simulink model "Pitch_Velocity_Controllers_Jetstar_FC4_Testing_Linear_Model"  (R2020a)
settings: Solver=FixedStepAuto  StartTime=0.0  StopTime=300  FixedStep=0.01  RelTol=1e-3
values from neighbouring files (symbols this model uses):
  A_Long = [Xu                     , Xw                      , -w_0                         , -g*cos(theta_0) ... (first row only)    [Longitudinal_Linearized_Matrices.m]
  B_Long = [Xdel_e                          , Xdel_t ... (first row only)    [Longitudinal_Linearized_Matrices.m]
  C_Long = eye(4)    [Longitudinal_Linearized_Matrices.m]
  D_Long = zeros(4,2)    [Longitudinal_Linearized_Matrices.m]
undefined symbols (not defined in the file or in its folder): theta_0, u_0, w_0, z_0
libraries: cstblocks x3, simulink_extras x1
settings Model: Creator=mohan  LastModifiedBy=mohan

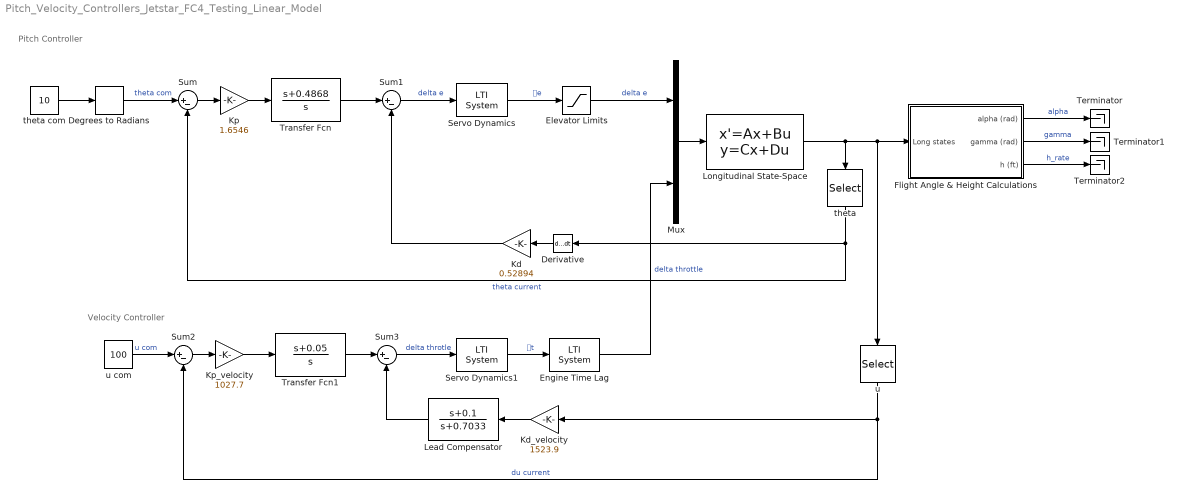
== system Pitch_Velocity_Controllers_Jetstar_FC4_Testing_Linear_Model ==
  note: Velocity Controller
  note: Pitch Controller
  Degrees to Radians : simulink_extras/Transformations/Degrees to Radians
  Derivative : Derivative
  Elevator Limits : Saturate  UpperLimit=25*pi/180  LowerLimit=-25*pi/180
  Engine Time Lag : cstblocks/LTI System  sys=tf(0.1,[1 0.1])  IC=[]
  Flight Angle & Height Calculations : Subsystem
  Kd : Gain  Gain=0.52894
  Kd_velocity : Gain  Gain=1523.9
  Kp : Gain  Gain=1.6546
  Kp_velocity : Gain  Gain=1027.7
  Lead Compensator : TransferFcn  Numerator=[1 0.1]  Denominator=[1 0.7033]
  Longitudinal State-Space : StateSpace  A=A_Long  B=B_Long  C=C_Long  D=D_Long  InitialCondition=[]
  Mux : Mux  Inputs=2
  Servo Dynamics : cstblocks/LTI System  sys=-tf(10,[1 10])  IC=[]
  Servo Dynamics1 : cstblocks/LTI System  sys=tf(10,[1 10])  IC=[]
  Sum{,1..3} (4 alike) : Sum  Inputs=|+-
  Terminator : Terminator
  Terminator1 : Terminator
  Terminator2 : Terminator
  Transfer Fcn : TransferFcn  Numerator=[1 0.4868]  Denominator=[1 0]
  Transfer Fcn1 : TransferFcn  Numerator=[1 0.05]  Denominator=[1 0]
  theta : Selector  InputPortWidth=4  IndexOptions=Index vector (dialog)  Indices=4  OutputSizes=1
  theta com : Constant  Value=10
  u : Selector  InputPortWidth=4  IndexOptions=Index vector (dialog)  Indices=1  OutputSizes=1
  u com : Constant  Value=100
  wires:
  Engine Time Lag/1 -> Mux/2  "delta throttle"
  theta/1 -> Sum/2, Derivative/1  "theta current"
  theta com/1 -> Degrees to Radians/1
  Longitudinal State-Space/1 -> Flight Angle & Height Calculations/1(Long states), u/1, theta/1
  Elevator Limits/1 -> Mux/1  "delta e"
  Derivative/1 -> Kd/1
  Transfer Fcn/1 -> Sum1/1
  Flight Angle & Height Calculations/3(h (ft)) -> Terminator2/1  "h_rate"
  Mux/1 -> Longitudinal State-Space/1
  Servo Dynamics/1 -> Elevator Limits/1  "𝛿e"
  Sum1/1 -> Servo Dynamics/1  "delta e"
  Kp/1 -> Transfer Fcn/1
  Sum/1 -> Kp/1
  Flight Angle & Height Calculations/2(gamma (rad)) -> Terminator1/1  "gamma"
  Kd/1 -> Sum1/2
  Degrees to Radians/1 -> Sum/1  "theta com"
  Flight Angle & Height Calculations/1(alpha (rad)) -> Terminator/1  "alpha"
  Sum3/1 -> Servo Dynamics1/1  "delta throtle"
  Transfer Fcn1/1 -> Sum3/1
  Servo Dynamics1/1 -> Engine Time Lag/1  "𝛿t"
  Kd_velocity/1 -> Lead Compensator/1
  Sum2/1 -> Kp_velocity/1
  Lead Compensator/1 -> Sum3/2
  Kp_velocity/1 -> Transfer Fcn1/1
  u com/1 -> Sum2/1  "u com"
  u/1 -> Kd_velocity/1, Sum2/2  "du current"

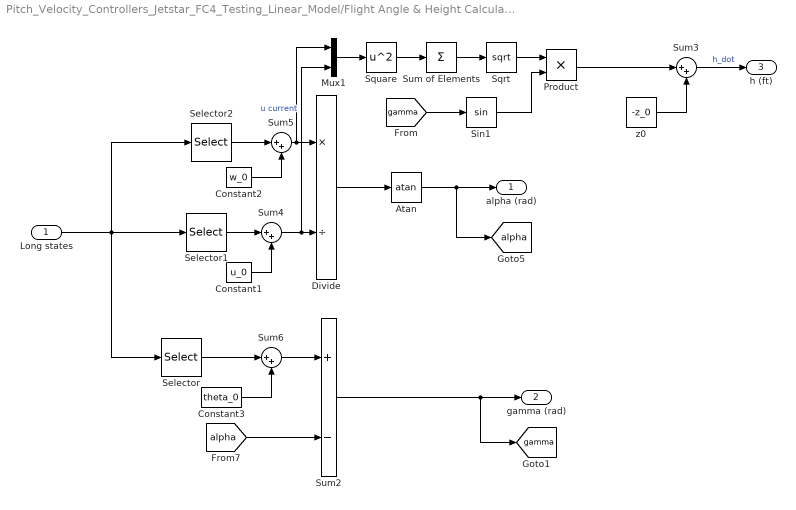
== system Pitch_Velocity_Controllers_Jetstar_FC4_Testing_Linear_Model/Flight Angle & Height Calculations ==
  Long states : Inport
  Atan : Trigonometry  Operator=atan
  Constant1 : Constant  Value=u_0
  Constant2 : Constant  Value=w_0
  Constant3 : Constant  Value=theta_0
  Divide : Product  Inputs=*/
  Mux1 : Mux  Inputs=2
  Product : Product
  Selector : Selector  InputPortWidth=4  IndexOptions=Index vector (dialog)  Indices=4  OutputSizes=1
  Selector1 : Selector  InputPortWidth=4  IndexOptions=Index vector (dialog)  Indices=1  OutputSizes=1
  Selector2 : Selector  InputPortWidth=4  IndexOptions=Index vector (dialog)  Indices=2  OutputSizes=1
  Sin1 : Trigonometry
  Sqrt : Sqrt  SaturateOnIntegerOverflow=on
  Square : Math  Operator=square  SaturateOnIntegerOverflow=on
  Sum of Elements : Sum  Inputs=+
  Sum2 : Sum  Inputs=+-
  Sum{3..6} (4 alike) : Sum  Inputs=|++
  z0 : Constant  Value=-z_0
  alpha (rad) : Outport
  gamma (rad) : Outport  Port=2
  h (ft) : Outport  Port=3
  tag scope: alpha=global, gamma=global
  wires:
  z0/1 -> Sum3/2
  Constant2/1 -> Sum5/2
  Sum2/1 -> [gamma], gamma (rad)/1
  Selector1/1 -> Sum4/1
  [gamma] -> Sin1/1
  Constant1/1 -> Sum4/2
  Atan/1 -> alpha (rad)/1, [alpha]
  Mux1/1 -> Square/1
  Square/1 -> Sum of Elements/1
  Sqrt/1 -> Product/1
  Constant3/1 -> Sum6/2
  Long states/1 -> Selector1/1, Selector2/1, Selector/1
  Sum4/1 -> Mux1/2, Divide/2  "u current"
  Sum3/1 -> h (ft)/1  "h_dot"
  Sum6/1 -> Sum2/1
  Sum5/1 -> Mux1/1, Divide/1
  Sum of Elements/1 -> Sqrt/1
  Selector2/1 -> Sum5/1
  [alpha] -> Sum2/2
  Sin1/1 -> Product/2
  Divide/1 -> Atan/1
  Selector/1 -> Sum6/1
  Product/1 -> Sum3/1
